simulink model "LQ_Guidance"  (R2016b)
settings: Solver=FixedStepAuto  StartTime=0.0  StopTime=tf  FixedStep=0.01  RelTol=1e-3
values from neighbouring files (symbols this model uses):
  k = k+1    (= 2)    [Nir_ref.m]
  R0 = eq2(t_1)    [P_1.m]
  rx_0 = r0*cos(lmbda_0)    [P_1.m]    (also in P_9_tgo_dlmbda.m)
  ry_0 = r0*sin(lmbda_0)    [P_1.m]    (also in P_9_tgo_dlmbda.m)
  Vc = r_norm./tgo_int    [Nir_ref.m]
undefined symbols (not defined in the file or in its folder): drx_0, dry_0
settings Model: Creator=Daniel  LastModifiedBy=Daniel

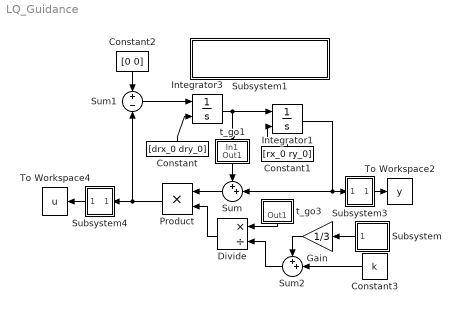
== system LQ_Guidance ==
  Constant : Constant  Value=[drx_0 dry_0]
  Constant1 : Constant  Value=[rx_0 ry_0]
  Constant2 : Constant  Value=[0 0]
  Constant3 : Constant  Value=k
  Divide : Product  Inputs=*/
  Gain : Gain  Gain=1/3
  Integrator1 : Integrator  InitialConditionSource=external  InitialCondition=Vc
  Integrator3 : Integrator  InitialConditionSource=external  InitialCondition=R0
  Product : Product
  Subsystem : Subsystem
  Subsystem1 : Subsystem
      mask Display: image('P_17_u.PNG');
  Subsystem3 : Subsystem
      mask Display: image('norm.PNG');
  Subsystem4 : Subsystem
      mask Display: image('norm.PNG');
  Sum : Sum  Inputs=++|
  Sum1 : Sum  Inputs=+|-
  Sum2 : Sum  Inputs=++|
  To Workspace2 : ToWorkspace  VariableName=y  SaveFormat=Timeseries  SampleTime=-1
  To Workspace4 : ToWorkspace  VariableName=u  SaveFormat=Timeseries  SampleTime=-1
  t_go1 : Subsystem
      mask Display: image('t_go_P.PNG');
  t_go3 : Subsystem
      mask Display: image('t_go_P.PNG');
  wires:
  Constant1/1 -> Integrator1/2
  Constant/1 -> Integrator3/2
  Product/1 -> Sum1/2, Subsystem4/1(In1)
  Sum1/1 -> Integrator3/1
  Constant2/1 -> Sum1/1
  Integrator3/1 -> t_go1/1(In1), Integrator1/1
  t_go3/1(Out1) -> Divide/1
  Sum2/1 -> Divide/2
  Subsystem/1(t_go^3) -> Gain/1
  Gain/1 -> Sum2/1
  Constant3/1 -> Sum2/2
  Divide/1 -> Product/2
  Subsystem4/1(Out1) -> To Workspace4/1
  Sum/1 -> Product/1
  t_go1/1(Out1) -> Sum/1
  Subsystem3/1(Out1) -> To Workspace2/1
  Integrator1/1 -> Sum/2, Subsystem3/1(In1)

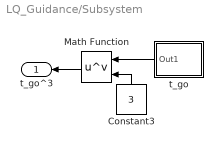
== system LQ_Guidance/Subsystem ==
  Constant3 : Constant  Value=3
  Math Function : Math  Operator=pow  SaturateOnIntegerOverflow=on
  t_go : Subsystem
  t_go^3 : Outport
  wires:
  t_go/1(Out1) -> Math Function/1
  Constant3/1 -> Math Function/2
  Math Function/1 -> t_go^3/1

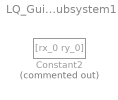
== system LQ_Guidance/Subsystem1 ==
  Constant2 : Constant  Commented=on  Value=[rx_0 ry_0]

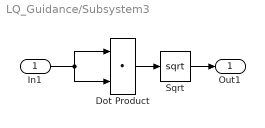
== system LQ_Guidance/Subsystem3 ==
  In1 : Inport
  Dot Product : DotProduct  InputSameDT=on  OutDataTypeStr=Inherit: Inherit via internal rule
  Sqrt : Sqrt  SaturateOnIntegerOverflow=on
  Out1 : Outport
  wires:
  Sqrt/1 -> Out1/1
  Dot Product/1 -> Sqrt/1
  In1/1 -> Dot Product/2, Dot Product/1

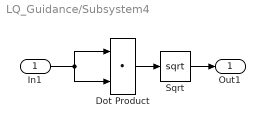
== system LQ_Guidance/Subsystem4 ==
  In1 : Inport
  Dot Product : DotProduct  InputSameDT=on  OutDataTypeStr=Inherit: Inherit via internal rule
  Sqrt : Sqrt  SaturateOnIntegerOverflow=on
  Out1 : Outport
  wires:
  Sqrt/1 -> Out1/1
  Dot Product/1 -> Sqrt/1
  In1/1 -> Dot Product/2, Dot Product/1

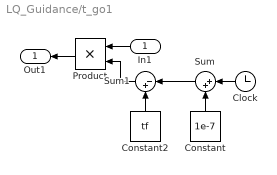
== system LQ_Guidance/t_go1 ==
  In1 : Inport
  Clock : Clock
  Constant : Constant  Value=1e-7
  Constant2 : Constant  Value=tf
  Product : Product
  Sum : Sum  Inputs=|++
  Sum1 : Sum  Inputs=|-+
  Out1 : Outport
  wires:
  Sum/1 -> Sum1/1
  Clock/1 -> Sum/1
  Sum1/1 -> Product/2
  Constant/1 -> Sum/2
  Constant2/1 -> Sum1/2
  In1/1 -> Product/1
  Product/1 -> Out1/1

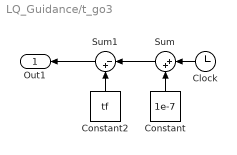
== system LQ_Guidance/t_go3 ==
  Clock : Clock
  Constant : Constant  Value=1e-7
  Constant2 : Constant  Value=tf
  Sum : Sum  Inputs=|++
  Sum1 : Sum  Inputs=|-+
  Out1 : Outport
  wires:
  Sum/1 -> Sum1/1
  Clock/1 -> Sum/1
  Constant/1 -> Sum/2
  Constant2/1 -> Sum1/2
  Sum1/1 -> Out1/1

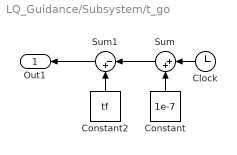
== system LQ_Guidance/Subsystem/t_go ==
  Clock : Clock
  Constant : Constant  Value=1e-7
  Constant2 : Constant  Value=tf
  Sum : Sum  Inputs=|++
  Sum1 : Sum  Inputs=|-+
  Out1 : Outport
  wires:
  Sum/1 -> Sum1/1
  Clock/1 -> Sum/1
  Sum1/1 -> Out1/1
  Constant/1 -> Sum/2
  Constant2/1 -> Sum1/2
